simulink model "Basic_DMT"  (R2014b)
settings: Solver=FixedStepDiscrete  SolverMode=SingleTasking  StartTime=0.0  StopTime=25e-6-14e-9*24  RelTol=1e-3
PreLoadFcn:
  | userName = getenv('UserName');
  | 
  | if strcmp(userName,'Tim')
  | cd C:\Users\Tim\Documents\GitHub\MA_1\Basic_DMT
  | else
  | cd C:\Users\Tim-UML\Documents\GitHub\MA_1\Basic_DMT
  | end
InitFcn:
  | userName = getenv('UserName');
  | 
  | if strcmp(userName,'Tim')
  | cd C:\Users\Tim\Documents\GitHub\MA_1\Basic_DMT
  | else
  | cd C:\Users\Tim-UML\Documents\GitHub\MA_1\Basic_DMT
  | end
values from neighbouring files (symbols this model uses):
  a0 = 0.21194908595403703    (= 0.211949085954)    [initScript.m]
  a1 = 0.576101828091926    (= 0.576101828092)    [initScript.m]
  a2 = a0    (= 0.211949085954)    [initScript.m]
  beta = 1    [initScript.m]
  bitPerSymb = 4    [initScript.m]
  chanDownFact = Tchan/SystemPeriod    [initScript.m]
  fftLen = 16    [initScript.m]
  fftLenActive = fftLenDMT    (= 32)    [initScript.m]
  fftLenDMT = 2*fftLen    (= 32)    [initScript.m]
  GI_Active = GI_LenDMT    (= 0)    [initScript.m]
  GI_Len = 0    [initScript.m]
  GI_LenDMT = 0    [initScript.m]
  M = log2(fftLen)    [initScript.m]
  sysgenSystemPeriod = 4e-9    (= 4e-09)    [initScript.m]
  SystemPeriod = 4e-9    (= 4e-09)    [initScript.m]
  upsampleFactor = 1    [initScript.m]
  usedSubCar = 14    [initScript.m]
undefined symbols (not defined in the file or in its folder): bitCount, get, modu_mode, Tb, Ts
libraries: xbsIndex_r4 x822, commdigbbndam3 x59, simulink x42, dspsigops x7, commrandsrc2 x6, dspbuff3 x4, dspxfrm3 x3, dspswit3 x2, commseqgen2 x1, dsparch4 x1, commutil2 x1, dspsnks4 x1
(part 10 of 10)

== system Basic_DMT/Sysgen_SIPaFFT/Guard_Interval/Rem_GI_DMT ==
  note: 11
  note: 11
  Re_In : Inport
  Im_In : Inport  Port=2
  Delay : xbsIndex_r4/Delay  rst=off  infoeditControl=Selection of Reset will increase slice count due to use of real FFs and instead of SRLs  en=off  latency=7  reg_retiming=off  dbl_ovrd=off  block_type=delay
  Delay1 : xbsIndex_r4/Delay  rst=off  infoeditControl=Selection of Reset will increase slice count due to use of real FFs and instead of SRLs  en=off  latency=7  reg_retiming=off  dbl_ovrd=off  block_type=delay
  Delay2 : xbsIndex_r4/Delay  rst=off  infoeditControl=Selection of Reset will increase slice count due to use of real FFs and instead of SRLs  en=off  latency=16  reg_retiming=off  dbl_ovrd=off  block_type=delay
  Delay3 : xbsIndex_r4/Delay  rst=off  infoeditControl=Selection of Reset will increase slice count due to use of real FFs and instead of SRLs  en=off  latency=16  reg_retiming=off  dbl_ovrd=off  block_type=delay
  Parallel to Serial : xbsIndex_r4/Parallel to Serial  output_order=Most Significant Word First  arith_type="Signed  (2's comp)"  output_bits=(bitCount+(log2(fftLen)+1))  bin_pt=fracLen  rst=off  en=off  latency=0  dbl_ovrd=off  block_type=p2s
      settings: infoedit=Each sample presented at the input becomes several samples presented serially at the output.
  Parallel to Serial1 : xbsIndex_r4/Parallel to Serial  output_order=Most Significant Word First  arith_type="Signed  (2's comp)"  output_bits=(bitCount+(log2(fftLen)+1))  bin_pt=fracLen  rst=off  en=off  latency=0  dbl_ovrd=off  block_type=p2s
      settings: infoedit=Each sample presented at the input becomes several samples presented serially at the output.
  Serial to Parallel : xbsIndex_r4/Serial to Parallel  input_order=Most Significant Word First  arith_type=Unsigned  output_bits=(bitCount+(log2(fftLen)+1))*(fftLenDMT+GI_LenDMT)  bin_pt=0  rst=off  en=off  latency=1  dbl_ovrd=off  block_type=s2p
      settings: infoedit=Groups of samples presented serially at the input become single samples presented at the output.
  Serial to Parallel1 : xbsIndex_r4/Serial to Parallel  input_order=Most Significant Word First  arith_type=Unsigned  output_bits=(bitCount+(log2(fftLen)+1))*(fftLenDMT+GI_LenDMT)  bin_pt=0  rst=off  en=off  latency=1  dbl_ovrd=off  block_type=s2p
      settings: infoedit=Groups of samples presented serially at the input become single samples presented at the output.
  Slice1 : xbsIndex_r4/Slice  nbits=(bitCount+(log2(fftLen)+1))*fftLenDMT  boolean_output=off  mode=Lower Bit Location + Width  bit1=0  base1=LSB of Input  bit0=0  base0=LSB of Input  dbl_ovrd=off  block_type=slice
  Slice16 : xbsIndex_r4/Slice  nbits=(bitCount+(log2(fftLen)+1))*fftLenDMT  boolean_output=off  mode=Lower Bit Location + Width  bit1=0  base1=LSB of Input  bit0=0  base0=LSB of Input  dbl_ovrd=off  block_type=slice
  Re : Outport
  Im : Outport  Port=2
  wires:
  Re_In/1 -> Delay/1
  Parallel to Serial/1 -> Delay2/1
  Delay/1 -> Serial to Parallel/1
  Serial to Parallel/1 -> Slice16/1
  Slice16/1 -> Parallel to Serial/1
  Delay2/1 -> Re/1
  Im_In/1 -> Delay1/1
  Parallel to Serial1/1 -> Delay3/1
  Delay1/1 -> Serial to Parallel1/1
  Serial to Parallel1/1 -> Slice1/1
  Slice1/1 -> Parallel to Serial1/1
  Delay3/1 -> Im/1

== system Basic_DMT/Sysgen_SIPaFFT/Guard_Interval/Rem_GI_OFDM ==
  note: 11
  Re_In : Inport
  Im_In : Inport  Port=2
  Delay2 : xbsIndex_r4/Delay  rst=off  infoeditControl=Selection of Reset will increase slice count due to use of real FFs and instead of SRLs  en=off  latency=7  reg_retiming=off  dbl_ovrd=off  block_type=delay
  Delay3 : xbsIndex_r4/Delay  rst=off  infoeditControl=Selection of Reset will increase slice count due to use of real FFs and instead of SRLs  en=off  latency=7  reg_retiming=off  dbl_ovrd=off  block_type=delay
  Parallel to Serial2 : xbsIndex_r4/Parallel to Serial  output_order=Most Significant Word First  arith_type="Signed  (2's comp)"  output_bits=(bitCount+(log2(fftLen)+1))  bin_pt=fracLen  rst=off  en=off  latency=0  dbl_ovrd=off  block_type=p2s
      settings: infoedit=Each sample presented at the input becomes several samples presented serially at the output.
  Parallel to Serial3 : xbsIndex_r4/Parallel to Serial  output_order=Most Significant Word First  arith_type="Signed  (2's comp)"  output_bits=(bitCount+(log2(fftLen)+1))  bin_pt=fracLen  rst=off  en=off  latency=0  dbl_ovrd=off  block_type=p2s
      settings: infoedit=Each sample presented at the input becomes several samples presented serially at the output.
  Serial to Parallel2 : xbsIndex_r4/Serial to Parallel  input_order=Most Significant Word First  arith_type=Unsigned  output_bits=(bitCount+(log2(fftLen)+1))*(fftLen+GI_Len)  bin_pt=0  rst=off  en=off  latency=1  dbl_ovrd=off  block_type=s2p
      settings: infoedit=Groups of samples presented serially at the input become single samples presented at the output.
  Serial to Parallel3 : xbsIndex_r4/Serial to Parallel  input_order=Most Significant Word First  arith_type=Unsigned  output_bits=(bitCount+(log2(fftLen)+1))*(fftLen+GI_Len)  bin_pt=0  rst=off  en=off  latency=1  dbl_ovrd=off  block_type=s2p
      settings: infoedit=Groups of samples presented serially at the input become single samples presented at the output.
  Slice17 : xbsIndex_r4/Slice  nbits=(bitCount+(log2(fftLen)+1))*fftLen  boolean_output=off  mode=Lower Bit Location + Width  bit1=0  base1=LSB of Input  bit0=0  base0=LSB of Input  dbl_ovrd=off  block_type=slice
  Slice18 : xbsIndex_r4/Slice  nbits=(bitCount+(log2(fftLen)+1))*fftLen  boolean_output=off  mode=Lower Bit Location + Width  bit1=0  base1=LSB of Input  bit0=0  base0=LSB of Input  dbl_ovrd=off  block_type=slice
  Re : Outport
  Im : Outport  Port=2
  wires:
  Parallel to Serial2/1 -> Re/1
  Parallel to Serial3/1 -> Im/1
  Slice18/1 -> Parallel to Serial2/1
  Delay2/1 -> Serial to Parallel2/1
  Delay3/1 -> Serial to Parallel3/1
  Serial to Parallel2/1 -> Slice18/1
  Slice17/1 -> Parallel to Serial3/1
  Serial to Parallel3/1 -> Slice17/1
  Re_In/1 -> Delay2/1
  Im_In/1 -> Delay3/1

== system Basic_DMT/Channel/Yes_Channel/Delay_upsample/Del_ups ==
  In1 : Inport
  Delay : Delay  DelayLength=upsampleFactor-grpDelayChannelFilt  InitialCondition=0
  Out1 : Outport
  wires:
  In1/1 -> Delay/1
  Delay/1 -> Out1/1

== system Basic_DMT/Channel/Yes_Channel/Delay_upsample/Delay_None ==
  In1 : Inport
  Out1 : Outport
  wires:
  In1/1 -> Out1/1

== system Basic_DMT/IFFTaPIS/Create_Frame_for_IFFT/OFDMorDMT/Frame_DMT ==
  note: Carrier 0 is set to 0 to prevent DC
      | Carrier N/2 is set to zero because
      |  this carrier is in the cutoff frequency of the filter
  Sub1 : Inport
  Sub2 : Inport  Port=2
  Sub3 : Inport  Port=3
  Sub4 : Inport  Port=4
  Sub5 : Inport  Port=5
  Sub6 : Inport  Port=6
  Sub7 : Inport  Port=7
  Sub8 : Inport  Port=8
  Sub9 : Inport  Port=9
  Sub10 : Inport  Port=10
  Sub11 : Inport  Port=11
  Sub12 : Inport  Port=12
  Sub13 : Inport  Port=13
  Sub14 : Inport  Port=14
  Complex to Real-Imag1 : ComplexToRealImag
  Complex to Real-Imag4 : ComplexToRealImag
  Constant : Constant  Value=0  OutDataTypeStr=double
  Math Function{1..14} (14 alike) : Math  Operator=conj  SaturateOnIntegerOverflow=on
  Mux1 : Mux  Inputs=32
  Real-Imag to Complex2 : RealImagToComplex
  Scope1 : Scope  Commented=on  NumInputPorts=4
      settings: YMin=-5~-5~-5~-5  YMax=5~5~5~5  SaveName=ScopeData63
  Unbuffer18 : Unbuffer  SampleBasedProcessing=Same as frame based
  Unbuffer19 : Unbuffer  SampleBasedProcessing=Same as frame based
  Out1 : Outport
  wires:
  Sub1/1 -> Math Function1/1, Mux1/2
  Sub2/1 -> Math Function2/1, Mux1/3
  Real-Imag to Complex2/1 -> Mux1/9, Mux1/1, Mux1/17, Mux1/25
  Math Function1/1 -> Mux1/32
  Constant/1 -> Real-Imag to Complex2/1, Real-Imag to Complex2/2
  Mux1/1 -> Complex to Real-Imag4/1, Out1/1
  Math Function3/1 -> Mux1/30
  Math Function2/1 -> Mux1/31
  Math Function5/1 -> Mux1/28
  Math Function4/1 -> Mux1/29
  Math Function7/1 -> Mux1/26
  Math Function6/1 -> Mux1/27
  Math Function9/1 -> Mux1/23
  Math Function8/1 -> Mux1/24
  Math Function11/1 -> Mux1/21
  Math Function10/1 -> Mux1/22
  Math Function13/1 -> Mux1/19
  Math Function12/1 -> Mux1/20
  Sub4/1 -> Math Function4/1, Mux1/5
  Sub6/1 -> Math Function6/1, Mux1/7
  Sub5/1 -> Math Function5/1, Mux1/6
  Sub7/1 -> Math Function7/1, Mux1/8
  Sub8/1 -> Math Function8/1, Mux1/10
  Sub11/1 -> Mux1/13, Math Function11/1
  Sub12/1 -> Math Function12/1, Mux1/14
  Sub13/1 -> Mux1/15, Math Function13/1
  Sub14/1 -> Mux1/16, Math Function14/1
  Sub9/1 -> Math Function9/1, Mux1/11
  Sub10/1 -> Math Function10/1, Mux1/12
  Math Function14/1 -> Mux1/18
  Unbuffer18/1 -> Scope1/1
  Complex to Real-Imag4/1 -> Unbuffer18/1
  Complex to Real-Imag4/2 -> Unbuffer19/1
  Unbuffer19/1 -> Scope1/2
  Complex to Real-Imag1/1 -> Scope1/3
  Complex to Real-Imag1/2 -> Scope1/4
  Sub3/1 -> Math Function3/1, Complex to Real-Imag1/1, Mux1/4

== system Basic_DMT/IFFTaPIS/Create_Frame_for_IFFT/OFDMorDMT/Frame_OFDM ==
  Sub1 : Inport
  Sub2 : Inport  Port=2
  Sub3 : Inport  Port=3
  Sub4 : Inport  Port=4
  Sub5 : Inport  Port=5
  Sub6 : Inport  Port=6
  Sub7 : Inport  Port=7
  Sub8 : Inport  Port=8
  Sub9 : Inport  Port=9
  Sub10 : Inport  Port=10
  Sub11 : Inport  Port=11
  Sub12 : Inport  Port=12
  Sub13 : Inport  Port=13
  Sub14 : Inport  Port=14
  Constant : Constant  Value=0  OutDataTypeStr=double
  Constant1 : Constant  Commented=on  Value=65555  SampleTime=Ts*fftLen
  Delay : Delay  Commented=on  DelayLength=1  InitialCondition=0
  Mux : Mux  Inputs=16
  Real-Imag to Complex : RealImagToComplex  Commented=on
  Real-Imag to Complex2 : RealImagToComplex
  Scope1 : Scope  Commented=on
      settings: SaveName=ScopeData46
  Subtract : Sum  Commented=on  Inputs=+-
  Upsample1 : dspsigops/Upsample  Commented=on  N=10  phase=0  RateOptions=Allow multirate processing  ic=0  mode=Unused parameter value
  Out1 : Outport
  wires:
  Mux/1 -> Out1/1
  Constant/1 -> Real-Imag to Complex2/1, Real-Imag to Complex2/2
  Constant1/1 -> Delay/1, Subtract/1
  Delay/1 -> Subtract/2
  Subtract/1 -> Real-Imag to Complex/2, Real-Imag to Complex/1, Scope1/1
  Real-Imag to Complex/1 -> Upsample1/1
  Real-Imag to Complex2/1 -> Mux/9, Mux/1
  Sub7/1 -> Mux/8
  Sub8/1 -> Mux/10
  Sub6/1 -> Mux/7
  Sub9/1 -> Mux/11
  Sub1/1 -> Mux/2
  Sub2/1 -> Mux/3
  Sub13/1 -> Mux/15
  Sub10/1 -> Mux/12
  Sub11/1 -> Mux/13
  Sub12/1 -> Mux/14
  Sub5/1 -> Mux/6
  Sub4/1 -> Mux/5
  Sub3/1 -> Mux/4
  Sub14/1 -> Mux/16

== system Basic_DMT/IFFTaPIS/Create_Frame_for_IFFT/OFDMorDMT/ImpulseResponse ==
  Sub1 : Inport
  Sub2 : Inport  Port=2
  Sub3 : Inport  Port=3
  Sub4 : Inport  Port=4
  Sub5 : Inport  Port=5
  Sub6 : Inport  Port=6
  Sub7 : Inport  Port=7
  Sub8 : Inport  Port=8
  Sub9 : Inport  Port=9
  Sub10 : Inport  Port=10
  Sub11 : Inport  Port=11
  Sub12 : Inport  Port=12
  Sub13 : Inport  Port=13
  Sub14 : Inport  Port=14
  Constant : Constant  Value=0  OutDataTypeStr=double
  Constant1 : Constant  Value=65555  SampleTime=Ts*usedSubCar*bitPerSymb
  Delay : Delay  DelayLength=1  InitialCondition=0
  Mux : Mux  Inputs=16
  Real-Imag to Complex : RealImagToComplex
  Real-Imag to Complex2 : RealImagToComplex
  Scope1 : Scope
      settings: SaveName=ScopeData46
  Subtract : Sum  Inputs=+-
  Terminator{,1..13} (14 alike) : Terminator
  Upsample1 : dspsigops/Upsample  Commented=on  N=10  phase=0  RateOptions=Allow multirate processing  ic=0  mode=Unused parameter value
  Out1 : Outport
  wires:
  Mux/1 -> Out1/1
  Constant/1 -> Real-Imag to Complex2/1, Real-Imag to Complex2/2
  Constant1/1 -> Delay/1, Subtract/1
  Delay/1 -> Subtract/2
  Subtract/1 -> Real-Imag to Complex/2, Real-Imag to Complex/1, Scope1/1
  Real-Imag to Complex/1 -> Mux/1
  Real-Imag to Complex2/1 -> Mux/2, Mux/3, Mux/4, Mux/5, Mux/6, Mux/7, Mux/8, Mux/16, Mux/15, Mux/14, Mux/13, Mux/12, Mux/11, Mux/10, Mux/9
  Sub2/1 -> Terminator1/1
  Sub1/1 -> Terminator/1
  Sub4/1 -> Terminator3/1
  Sub3/1 -> Terminator2/1
  Sub6/1 -> Terminator5/1
  Sub5/1 -> Terminator4/1
  Sub7/1 -> Terminator6/1
  Sub9/1 -> Terminator8/1
  Sub8/1 -> Terminator7/1
  Sub11/1 -> Terminator10/1
  Sub10/1 -> Terminator9/1
  Sub13/1 -> Terminator12/1
  Sub12/1 -> Terminator11/1
  Sub14/1 -> Terminator13/1

== matlab function Basic_DMT/Total Bits // Subchannel Information/Total-Bits  ==
  data: y output; x input
function y = fcn(x)
%#codegen
%Total-Bits
%Total number of Bits in all channels
y=sum(x)

end

== matlab function Basic_DMT/Total Bits // Subchannel Information/Sub-Channel-Information ==
  data: y output
function y = fcn()
%#codegen
%Sub-Channel-Information
%Number of Bits per Channel

y=zeros(2,1);
y(1) = 8;
y(2) = 6;

end

== matlab function Basic_DMT/SIP /MATLAB Function ==
  data: num input; sel output; push output; pop output; k data_store_memory; state data_store_memory; loopCount data_store_memory; usedSubCar parameter; bitPerSymb parameter; subCar data_store_memory; fftLen parameter
function [sel,push,pop] = simu_fsm_subc_alloc(num, usedSubCar, bitPerSymb, fftLen)
%aasdas
global state;
global k;
global loopCount;
global subCar;

%ProcessingFrequency divided by the Bit Frequency
freqDivider = 5;
if loopCount == 1
    A=1;
else
    A=0;
end
loopCount = loopCount +1;
if loopCount >= freqDivider
    loopCount = 0;
end  

if loopCount >= bitPerSymb 
subCar = subCar + 1;
end
if subCar >= fftLen
    subCar=1;
end

if subCar == 1 || subCar == 8
    B=1;
else
    B=0;
end

if (state == 0 || state == 2)  
    k=0;
end
if (state == 1 || state == 3) 
    k=k+1;
end


if num > (usedSubCar*bitPerSymb)-1
    X=1;
else
    X=0;
end

if  k>= (usedSubCar*bitPerSymb)
    Y=1;
else
    Y=0;
end


switch state
    case 0
        sel = 0;
        pop = 0;
        push=0;
        if X
            if A
                state=3;
            else
                state = 1;
            end
        else
            if A
                state=2;
            else
                state = 0;
            end
        end
    case 1
        
        sel = 1;
        pop = 1;
        push= 0;
        if Y
            if A 
            state=2;
            else
                state=0;
            end
        else
            if A
            state=3;
            else
                state=1;
            end
        end
        
  case 2
    sel = 0;
    pop = 0;
    push = 1;
    if X
        if A
            state=3;
        else
            state = 1;
        end
    else
        if A
            state=2;
        else
            state = 0;
        end
    end  
  case 3
        sel = 1;
        pop = 1;
        push= 1;
        if Y
            if A
            state=2;
            else
                state=0;
            end
        else
            if A
            state=3;
            else
                state=1;
            end
        end
    otherwise  
        sel = 0;
        pop = 0;
        push = 0;
end
end

== matlab function Basic_DMT/IFFTaPIS/MATLAB Function ==
  data: push_en input; push output; pop output; state data_store_memory; loopCount data_store_memory; k data_store_memory; fftLenActive parameter; GI_Active parameter; chanDownFact parameter
function [push,pop] = simu_fsm_bef_chan (  push_en, fftLenActive, GI_Active, chanDownFact)

global state;
global loopCount;
global k;

if loopCount == 0
    Y = 1;
else
    Y = 0;
end

loopCount = loopCount +1;
if loopCount >= chanDownFact
    loopCount = 0;
end    

% X = (k<= (fftLenActive+ GI_Active-1));
% k=k+1;
% 
% if k >= (fftLenActive+ GI_Active) *5
%     k=0;
% end
if push_en
    X=1;
else
    X=0;
end


switch state
    case 0
        pop = 0;
        push=1;
        if X
            if Y
                state = 1;
            else
                state = 0;
            end
            
        else           
            if Y
                state = 2;
            else
               state = 3;
            end   
        end
        
    case 1
        pop = 1;
        push= 1;       
        if X
            if Y
                state = 1;
            else
                state = 0;
            end
            
        else           
            if Y
                state = 2;
            else
                state = 3;
            end   
        end
    case 2
        pop = 1;
        push= 0;       
        if X
            if Y
                state = 1;
            else
                state = 0;
            end
            
        else           
            if Y
                state = 2;
            else
                state = 3;
            end   
        end
         case 3
        pop = 0;
        push= 0;       
        if X
            if Y
                state = 1;
            else
                state = 0;
            end
            
        else           
            if Y
                state = 2;
            else
                state = 3;
            end   
        end
    otherwise
        pop = 0;
        push= 0;   
end
end

== matlab function Basic_DMT/IFFTaPIS/Guard_Interval/Set_GI_OFDM/MATLAB Function ==
  data: inp input; i1 input; out output; o1 output; o2 output; o3 output; o4 output; o5 output; o6 output; o7 output; o8 output; o9 output; o10 output; o11 output; o12 output; o13 output; o14 output; o15 output; o16 output; pop output; k data_store_memory; state data_store_memory; loopCount data_store_memory; i2 input; i3 input; i4 input; i5 input; i6 input; i7 input; i8 input; i9 input; i10 input; i11 input; i12 input; i13 input; i14 input; i15 input; i16 input
function [out, o1 , o2 , o3 , o4 , o5 , o6 , o7 , o8 , o9 , o10, o11, o12, ...
               o13, o14, o15, o16, pop] = simu_fsm_GI_OFDM(...
          inp, i1 , i2 , i3 , i4 , i5 , i6 , i7 , i8 , i9 , i10, i11, i12, ...
               i13, i14, i15, i16)
%aasdas
global state;
% global k;
global loopCount;

%ProcessingFrequency divided by the Bit Frequency
% freqDivider = 5;
% if loopCount == 1
%     A=1;
% else
%     A=0;
% end
loopCount = loopCount +1;
if loopCount >= 16*5
    loopCount = 0;
end    

o1=i1;
o2=i2;
o3=i3;
o4=i4;
o5=i5;
o6=i6;
o7=i7;
o8=i8;
o9=i9;
o10=i10;
o11=i11;
o12=i12;
o13=i13;
o14=i14;
o15=i15;
o16=i16;
pop = 0;
out = 0;
switch state
    case 0       
        if loopCount == 1            
            state=1;           
        else
            state=0;            
        end
        
    case 1%Input
        o1=inp;
        state=2;       
    case 2
        o2=inp;
        state=3;
    case 3
        o3=inp;
        state=4;
    case 4
        o4=inp;
        state=5;
    case 5
        o5=inp;
        state=6;
    case 6
        o6=inp;
        state=7;
    case 7
        o7=inp;
        state=8;
    case 8
        o8=inp;
        state=9;
    case 9
        o9=inp;
        state=10;
    case 10
        o10=inp;
        state=11;
    case 11
        o11=inp;
        state=12;
    case 12
        o12=inp;
        state=13;
    case 13
        o13=inp;
        state=14;
    case 14
        o14=inp;
        state=15;
    case 15
        o15=inp;
        state=16;
    case 16
        o16=inp;
        state=17;
    case 17%Output prefix
        out=i13;
        pop=1;
        state=18;
    case 18
        out=i14;
        pop=1;
        state=19;
    case 19
        out=i15;
        pop=1;
        state=20;
    case 20
        out=i16;
        pop=1;
        state=21;
    case 21%Output Data
        out=i1;
        pop=1;
        state=22;
    case 22
        out=i2;
        pop=1;
        state=23;
    case 23
        out=i3;
        pop=1;
        state=24;
    case 24
        out=i4;
        pop=1;
        state=25;
    case 25
        out=i5;
        pop=1;
        state=26;
    case 26
        out=i6;
        pop=1;
        state=27;
    case 27
        out=i7;
        pop=1;
        state=28;
    case 28
        out=i8;
        pop=1;
        state=29;
    case 29
        out=i9;
        pop=1;
        state=30;
    case 30
        out=i10;
        pop=1;
        state=31;
    case 31
        out=i11;
        pop=1;
        state=32;
    case 32
        out=i12;
        pop=1;
        state=33;
    case 33
        out=i13;
        pop=1;
        state=34;
    case 34
        out=i14;
        pop=1;
        state=35;
    case 35
        out=i15;
        pop=1;
        state=36;
    case 36
        out=i16;
        pop=1;
        state=0;
end
end

== matlab function Basic_DMT/IFFTaPIS/Guard_Interval/None/MATLAB Function ==
  data: push_en output; k data_store_memory; fftLenActive parameter
function push_en   = simu_fsm_NO_GI (  fftLenActive)

global k;


push_en = (k<= (fftLenActive-1));
k=k+1;

if k >= (fftLenActive) *5
    k=0;
end


end

== matlab function Basic_DMT/SIPaFFT/MATLAB Function ==
  data: num input; sel output; push output; pop output; k data_store_memory; state data_store_memory; loopCount data_store_memory; GI_Active parameter; fftLenActive parameter
function [sel,push,pop] = simu_fsm_recv_inp(num, GI_Active, fftLenActive)
%aasdas
global state;
global k;
global loopCount;

%ProcessingFrequency divided by the Bit Frequency
freqDivider = 14;
if loopCount == 1
    A=1;
else
    A=0;
end
loopCount = loopCount +1;
if loopCount >= freqDivider
    loopCount = 0;
end    
switch state
    case 0
        k=0;
        sel = 0;
        pop = 0;
        push=0;
        if num > (GI_Active+fftLenActive)-1
            if A
                state=3;
            else
                state = 1;
            end
        else
            if A
                state=2;
            else
                state = 0;
            end
        end
        
    case 1
        k=k+1;
        sel = 1;
        pop = 1;
        push= 0;
        if k>= (GI_Active+fftLenActive)
            if A
            state=2;
            else
                state=0;
            end
        else
            if A
            state=3;
            else
                state=1;
            end
        end
        
  case 2
    k=0;
    sel = 0;
    pop = 0;
    push = 1;
    if num > (GI_Active+fftLenActive)-1
        if A
            state=3;
        else
            state = 1;
        end
    else
        if A
            state=2;
        else
            state = 0;
        end
    end  
  case 3
        k=k+1;
        sel = 1;
        pop = 1;
        push= 1;
        if k>= (GI_Active+fftLenActive)
            if A
            state=2;
            else
                state=0;
            end
        else
            if A
            state=3;
            else
                state=1;
            end
        end
    otherwise  
        sel = 0;
        pop = 0;
        push = 0;
end
end

== matlab function Basic_DMT/IFFTaPIS/FSM_FIFO/MATLAB Function1 ==
  data: num input; sel output; push output; pop output; k data_store_memory; state data_store_memory; loopCount data_store_memory; fftLenActive parameter
function [sel,push,pop] = simu_fsm_bef_IFFT(num, fftLenActive)
%aasdas
global state;
global k;
global loopCount;

%Transistion from 14e-9 to 4e-9
if loopCount == 0 && k==0
    Y=1;
    k=1;
else
    Y=0;    
end

if loopCount == 0 && k==1
    Z=1;
    k=0;
else
    Z=0;    
end

loopCount = loopCount +1;

if loopCount == 4 && k==1
    loopCount = 0;
end    
if loopCount == 3 && k==0
    loopCount = 0;
end 

if num >= fftLenActive
    X=1;
else
    X=0;
end
switch state
    case 0
        sel = 0;
        pop = 0;
        push= 0;
        if X
            if Y
                if Z
                disp('error');
                else
                state = 4;
                end
            else
                if Z
                 disp('error');
                else
                state = 3;
                end
            end
        else
             if Y
                if Z
                disp('error');
                else
                state = 1;
                end
            else
                if Z
                 disp('error');
                else
                state=0;
                end
            end
        end
        
    case 1
        sel = 0;
        pop = 0;
        push= 1;
        if X
            if Y
                if Z
                disp('error');
                else
                state = 4;
                end
            else
                if Z
                 disp('error');
                else
                state = 3;
                end
            end
        else
             if Y
                if Z
                disp('error');
                else
                state = 1;
                end
            else
                if Z
                 disp('error');
                else
                state=0;
                end
            end
        end
        
  case 2
        sel = 0;
        pop = 1;
        push= 1;
        if X
            if Y
                if Z
                disp('error');
                else
                state = 4;
                end
            else
                if Z
                 disp('error');
                else
                state = 3;
                end
            end
        else
             if Y
                if Z
                disp('error');
                else
                state = 1;
                end
            else
                if Z
                 disp('error');
                else
                state=0;
                end
            end
        end
  case 3
        sel = 1;
        pop = 1;
        push= 1;
        if X
            if Y
                if Z
                disp('error');
                else
                state = 4;
                end
            else
                if Z
                 disp('error');
                else
                state = 3;
                end
            end
        else
             if Y
                if Z
                disp('error');
                else
                state = 1;
                end
            else
                if Z
                 disp('error');
                else
                state=0;
                end
            end
        end
    otherwise  
        sel = 0;
        pop = 0;
        push = 0;
end
end
